simulink model "discretizacion_ZOH_retardo_mayor"  (R2018a)
settings: Solver=VariableStepAuto  StartTime=0.0  StopTime=10.0  RelTol=1e-3
settings Model: Creator=pablo  LastModifiedBy=pablo

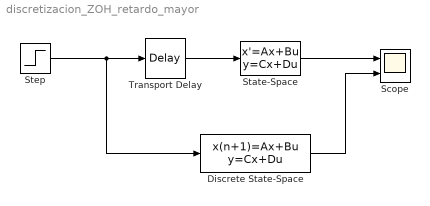
== system discretizacion_ZOH_retardo_mayor ==
  Discrete State-Space : DiscreteStateSpace  A=[0.37 0.24 0.39 0;0 0 1 0; 0 0 0 1;0 0 0 0]  B=[0 0 0 1]'  C=eye(4)  D=zeros(4,1)  InitialCondition=[0,0,0,0]'
  Scope : Scope  NumInputPorts=2
  State-Space : StateSpace  A=-1  D=0  InitialCondition=0
  Step : Step  SampleTime=0
  Transport Delay : TransportDelay  DelayTime=2.5
  wires:
  Step/1 -> Discrete State-Space/1, Transport Delay/1
  Transport Delay/1 -> State-Space/1
  State-Space/1 -> Scope/1
  Discrete State-Space/1 -> Scope/2
